simulink model "Metodo_NQ"  (R2023a)
settings: Solver=VariableStepAuto  StartTime=0.0  StopTime=200  RelTol=1e-3
libraries: cstblocks x3
settings Model: Creator=mayber  LastModifiedBy=mayber

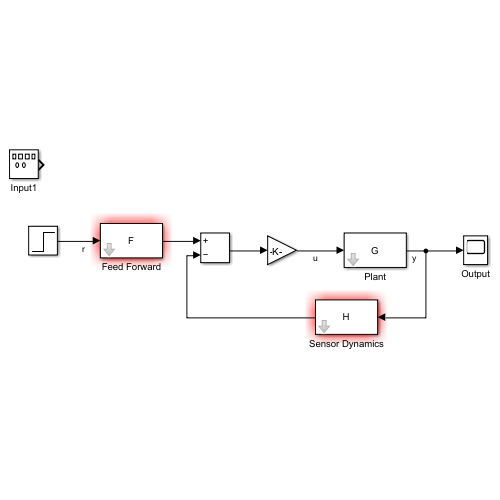
[thumbnail: Simulink's stored preview of the top-level diagram]
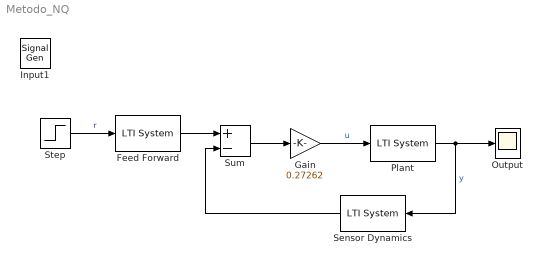
== system Metodo_NQ ==
  Feed Forward : cstblocks/LTI System  sys=F  IC=[]
  Gain : Gain  Gain=0.27262
  Input1 : SignalGenerator
  Output : Scope
  Plant : cstblocks/LTI System  sys=G  IC=[]
  Sensor Dynamics : cstblocks/LTI System  sys=H  IC=[]
  Step : Step  SampleTime=0
  Sum : Sum  Inputs=+-
  wires:
  Step/1 -> Feed Forward/1  "r"
  Feed Forward/1 -> Sum/1
  Sensor Dynamics/1 -> Sum/2
  Sum/1 -> Gain/1
  Gain/1 -> Plant/1  "u"
  Plant/1 -> Output/1, Sensor Dynamics/1  "y"
